simulink model "uz_threephase_VSD_transformation"  (R2021b)
settings: Solver=FixedStepAuto  StartTime=0.0  StopTime=inf  RelTol=1e-3
libraries: hdlsllib x1
settings Model: DataTypeOverride=Off  Creator=ts  LastModifiedBy=valen
settings SolverCC: AlgebraicLoopSolver=TrustRegion  AutoInsertRateTranBlk=on
settings DataIOCC: LimitDataPoints=on  SaveOutput=off  SaveTime=off
settings OptimizationCC: BlockReduction=off  ConditionallyExecuteInputs=off  DefaultParameterBehavior=Inlined  InheritOutputTypeSmallerThanSingle=on  LifeSpan=inf
settings DebuggingCC: AlgebraicLoopMsg=error  SingleTaskRateTransMsg=error  AllowSymbolicDim=off  StrictBusMsg=ErrorOnBusTreatedAsVector  SFUnexpectedBacktrackingDiag=warning  SFNoUnconditionalDefaultTransitionDiag=warning  SFExecutionAtInitializationDiag=none  SFMachineParentedDataDiag=warning  ArithmeticOperatorsInVariantConditions=warning
settings HardwareCC: ProdBitPerPointer=32  ProdBitPerSizeT=32  ProdBitPerPtrDiffT=32  ProdLargestAtomicFloat=None  ProdIntDivRoundTo=Undefined  ProdEndianess=Unspecified  ProdWordSize=32  ProdHWDeviceType=ASIC/FPGA->ASIC/FPGA  ProdEqTarget=off
settings SFSimCC: SimUseLocalCustomCode=off  CustomCodeUndefinedFunction=UseInterfaceOnly
settings RTWCC: RTWUseLocalCustomCode=off
settings CodeAppCC: StateflowObjectComments=on
settings GRTTargetCC: TargetLangStandard=C89/C90 (ANSI)
settings ConfigComp: CovScope=ReferencedModels  CovMetricSettings=dw  CovSaveCumulativeToWorkspaceVar=on  CovSaveSingleToWorkspaceVar=on  CovExternalEMLEnable=off  CovSFcnEnable=off

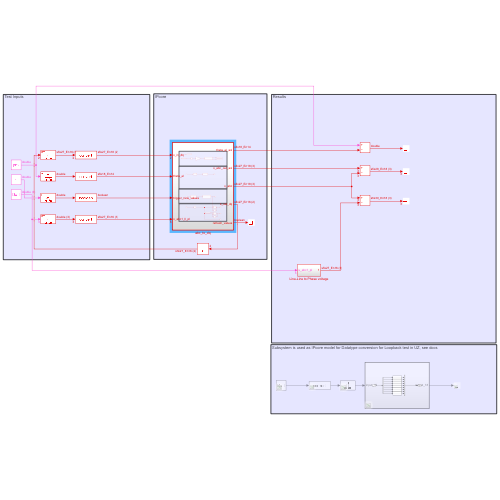
[thumbnail: Simulink's stored preview of the top-level diagram]
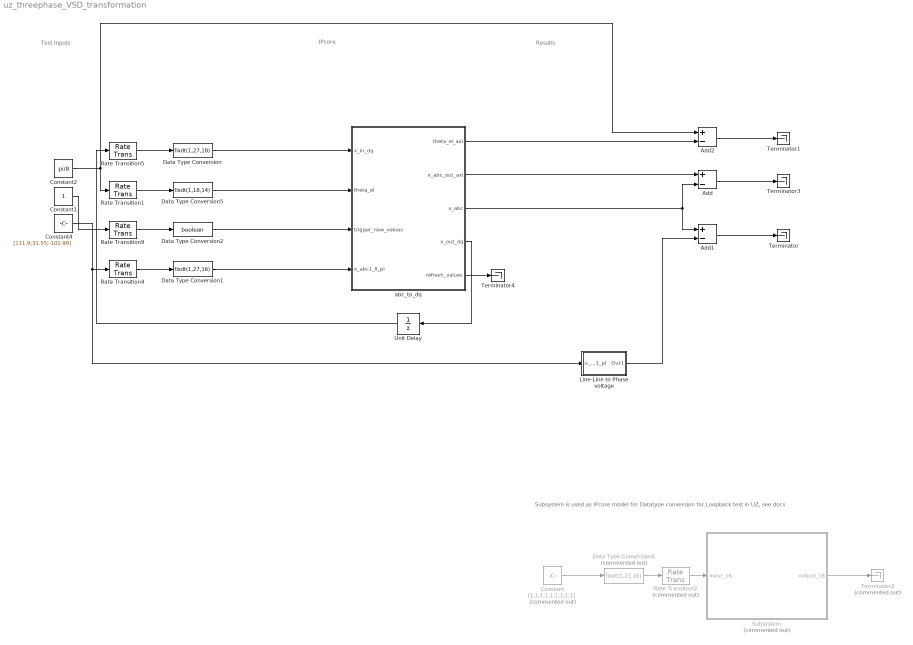
== system uz_threephase_VSD_transformation ==
  note: Subsystem is used as IPcore model for Datatype conversion for Loopback test in UZ, see docs
  note: Results
  note: Test Inputs
  note: IPcore
  Add : Sum  Inputs=+-
  Add1 : Sum  Inputs=+-
  Add2 : Sum  Inputs=+-
  Constant : Constant  Commented=on  Value=[1;1;1;1;1;1;1;1;1]
  Constant1 : Constant
  Constant2 : Constant  Value=pi/8
  Constant4 : Constant  Value=[111.9;31.55;-101.99]
  Data Type Conversion : DataTypeConversion  OutDataTypeStr=fixdt(1,27,18)
  Data Type Conversion1 : DataTypeConversion  OutDataTypeStr=fixdt(1,27,16)
  Data Type Conversion2 : DataTypeConversion  OutDataTypeStr=boolean
  Data Type Conversion5 : DataTypeConversion  OutDataTypeStr=fixdt(1,18,14)
  Data Type Conversion6 : DataTypeConversion  Commented=on  OutDataTypeStr=fixdt(1,27,16)
  Line-Line to Phase voltage : Subsystem
  Rate Transition{1,4..5,9} (4 alike) : RateTransition  OutPortSampleTime=ts_uz_ninephase_VSD_transformation
  Rate Transition2 : RateTransition  Commented=on  OutPortSampleTime=ts_uz_ninephase_VSD_transformation
  Subsystem : Subsystem  Commented=on  TreatAsAtomicUnit=on
  Terminator{,1,3..4} (4 alike) : Terminator
  Terminator2 : Terminator  Commented=on
  Unit Delay : UnitDelay  SampleTime=-1  HasFrameUpgradeWarning=on
  abc_to_dq : Subsystem  TreatAsAtomicUnit=on
  wires:
  Data Type Conversion/1 -> abc_to_dq/1(x_in_dq)
  Data Type Conversion1/1 -> abc_to_dq/4(x_abc1_ll_pl)
  Rate Transition5/1 -> Data Type Conversion/1
  Rate Transition4/1 -> Data Type Conversion1/1
  Data Type Conversion2/1 -> abc_to_dq/3(trigger_new_values)
  Rate Transition9/1 -> Data Type Conversion2/1
  Constant1/1 -> Rate Transition9/1
  Data Type Conversion5/1 -> abc_to_dq/2(theta_el)
  Rate Transition1/1 -> Data Type Conversion5/1
  abc_to_dq/4(x_out_dq) -> Unit Delay/1
  Constant2/1 -> Add2/1, Rate Transition1/1
  abc_to_dq/3(x_abc) -> Add1/1, Add/2
  abc_to_dq/2(x_abc_out_axi) -> Add/1
  Add1/1 -> Terminator/1
  abc_to_dq/1(theta_el_axi) -> Add2/2
  Add2/1 -> Terminator1/1
  Constant4/1 -> Line-Line to Phase voltage/1(u_abc1_pl), Rate Transition4/1
  Add/1 -> Terminator3/1
  Unit Delay/1 -> Rate Transition5/1
  Line-Line to Phase voltage/1(Out1) -> Add1/2
  Subsystem/1(output_18) -> Terminator2/1
  Constant/1 -> Data Type Conversion6/1
  Data Type Conversion6/1 -> Rate Transition2/1
  Rate Transition2/1 -> Subsystem/1(input_16)
  abc_to_dq/5(refresh_values) -> Terminator4/1

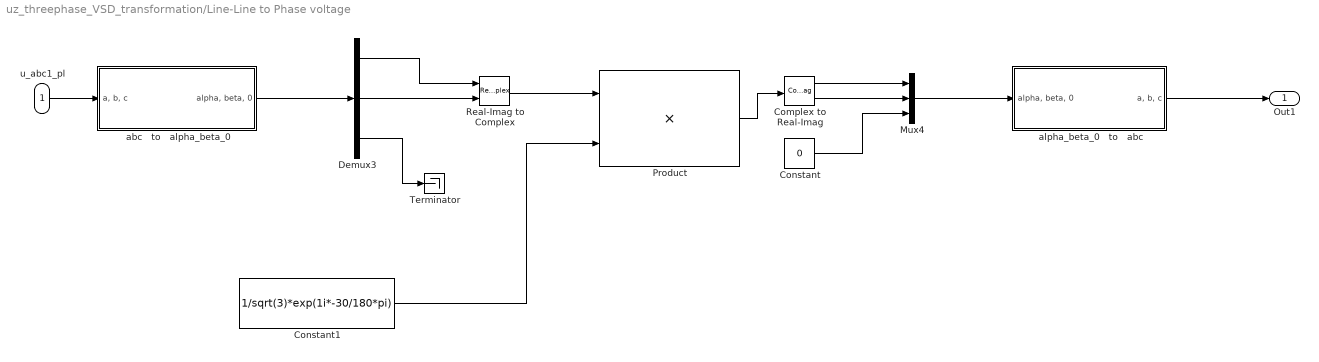
== system uz_threephase_VSD_transformation/Line-Line to Phase voltage ==
  u_abc1_pl : Inport
  Complex to Real-Imag : ComplexToRealImag
  Constant : Constant  Value=0  OutDataTypeStr=fixdt(1,27,16)  SampleTime=-1
  Constant1 : Constant  Value=1/sqrt(3)*exp(1i*-30/180*pi)  OutDataTypeStr=fixdt(1,18,16)  SampleTime=-1
  Demux3 : Demux  Outputs=3
  Mux4 : Mux  Inputs=3
  Product : Product  OutDataTypeStr=fixdt(1,27,16)
  Real-Imag to Complex : RealImagToComplex
  Terminator : Terminator
  abc   to   alpha_beta_0 : Subsystem
  alpha_beta_0   to   abc : Subsystem
  Out1 : Outport
  wires:
  Demux3/2 -> Real-Imag to Complex/2
  Complex to Real-Imag/1 -> Mux4/1
  Mux4/1 -> alpha_beta_0   to   abc/1("alpha, beta, 0  ")
  Product/1 -> Complex to Real-Imag/1
  Real-Imag to Complex/1 -> Product/1
  Demux3/1 -> Real-Imag to Complex/1
  Complex to Real-Imag/2 -> Mux4/2
  Constant/1 -> Mux4/3
  u_abc1_pl/1 -> abc   to   alpha_beta_0/1("a, b, c")
  Demux3/3 -> Terminator/1
  abc   to   alpha_beta_0/1("alpha, beta, 0 ") -> Demux3/1
  alpha_beta_0   to   abc/1("a, b, c") -> Out1/1
  Constant1/1 -> Product/2

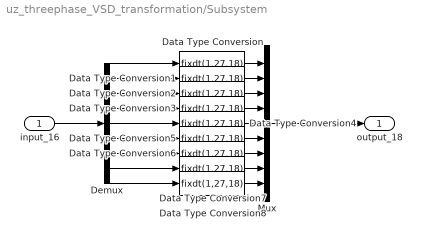
== system uz_threephase_VSD_transformation/Subsystem ==
  input_16 : Inport
  Data Type Conversion{,1..8} (9 alike) : DataTypeConversion  OutDataTypeStr=fixdt(1,27,18)
  Demux : Demux  Outputs=9
  Mux : Mux  Inputs=9
  output_18 : Outport
  wires:
  input_16/1 -> Demux/1
  Demux/1 -> Data Type Conversion/1
  Demux/2 -> Data Type Conversion1/1
  Demux/3 -> Data Type Conversion2/1
  Demux/6 -> Data Type Conversion5/1
  Demux/5 -> Data Type Conversion4/1
  Demux/4 -> Data Type Conversion3/1
  Demux/7 -> Data Type Conversion6/1
  Demux/8 -> Data Type Conversion7/1
  Demux/9 -> Data Type Conversion8/1
  Data Type Conversion/1 -> Mux/1
  Data Type Conversion1/1 -> Mux/2
  Data Type Conversion2/1 -> Mux/3
  Data Type Conversion3/1 -> Mux/4
  Data Type Conversion4/1 -> Mux/5
  Data Type Conversion5/1 -> Mux/6
  Data Type Conversion6/1 -> Mux/7
  Data Type Conversion7/1 -> Mux/8
  Data Type Conversion8/1 -> Mux/9
  Mux/1 -> output_18/1

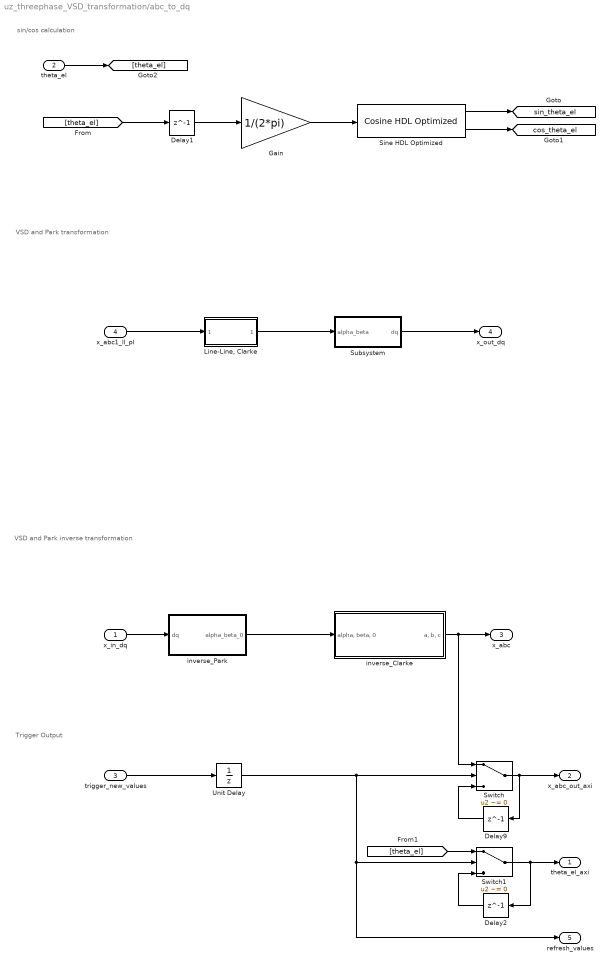
== system uz_threephase_VSD_transformation/abc_to_dq ==
  note: Trigger Output
  note: VSD and Park inverse transformation
  note: VSD and Park transformation
  note: sin/cos calculation
  x_in_dq : Inport
  theta_el : Inport  Port=2
  trigger_new_values : Inport  Port=3
  x_abc1_ll_pl : Inport  Port=4
  Delay1 : Delay  DelayLength=1
  Delay2 : Delay  DelayLength=1
  Delay9 : Delay  DelayLength=1
  Gain : Gain  Gain=1/(2*pi)  OutDataTypeStr=fixdt(1,18,16)
  "Line-Line, Clarke" : Subsystem
  Sine HDL Optimized : hdlsllib/Lookup Tables/Cosine HDL Optimized  OutputFormula=sin(2*pi*u) and cos(2*pi*u)  NumDataPoints=256  TableDataTypeStr=fixdt(0,17,16)  SimulateLUTROMDelay=off
      settings: SourceProductBaseCode=SL
  Subsystem : Subsystem
  Switch : Switch  Criteria=u2 ~= 0
  Switch1 : Switch  Criteria=u2 ~= 0
  Unit Delay : UnitDelay  SampleTime=-1  HasFrameUpgradeWarning=on
  inverse_Clarke : Subsystem
  inverse_Park : Subsystem
  theta_el_axi : Outport
  x_abc_out_axi : Outport  Port=2
  x_abc : Outport  Port=3
  x_out_dq : Outport  Port=4
  refresh_values : Outport  Port=5
  tag scope: cos_theta_el=global, sin_theta_el=global
  wires:
  "Line-Line, Clarke"/1(alpha_beta) -> Subsystem/1(alpha_beta)
  Delay9/1 -> Switch/3
  trigger_new_values/1 -> Unit Delay/1
  Switch/1 -> x_abc_out_axi/1, Delay9/1
  Delay1/1 -> Gain/1
  x_abc1_ll_pl/1 -> "Line-Line, Clarke"/1(u_abc1_pl)
  Gain/1 -> Sine HDL Optimized/1
  Sine HDL Optimized/1 -> [sin_theta_el]
  Sine HDL Optimized/2 -> [cos_theta_el]
  Delay2/1 -> Switch1/3
  Switch1/1 -> theta_el_axi/1, Delay2/1
  Unit Delay/1 -> refresh_values/1, Switch1/2, Switch/2
  Subsystem/1(dq) -> x_out_dq/1
  theta_el/1 -> [theta_el]
  [theta_el] -> Delay1/1
  [theta_el] -> Switch1/1
  inverse_Park/1(alpha_beta_0) -> inverse_Clarke/1("alpha, beta, 0  ")
  x_in_dq/1 -> inverse_Park/1(dq)
  inverse_Clarke/1("a, b, c") -> Switch/1, x_abc/1

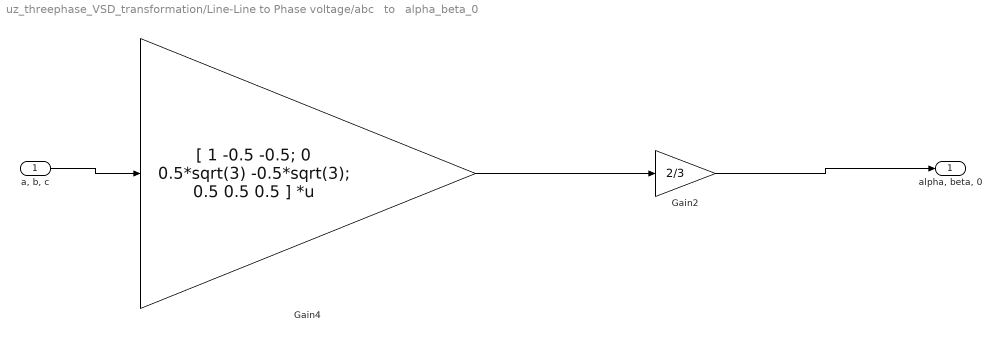
== system uz_threephase_VSD_transformation/Line-Line to Phase voltage/abc   to   alpha_beta_0 ==
  "a, b, c" : Inport  PortDimensions=3
  Gain2 : Gain  Gain=2/3  ParamDataTypeStr=fixdt(1,18,16)  SaturateOnIntegerOverflow=on  OutDataTypeStr=Inherit: Same as input
  Gain4 : Gain  Gain="[ 1   -0.5   -0.5; 0   0.5*sqrt(3)   -0.5*sqrt(3); 0.5  0.5  0.5 ]"  Multiplication=Matrix(K*u) (u vector)  ParamDataTypeStr=fixdt(1,18,16)  OutDataTypeStr=fixdt(1,27,16)  SaturateOnIntegerOverflow=on
  "alpha, beta, 0 " : Outport
  wires:
  Gain2/1 -> "alpha, beta, 0 "/1
  "a, b, c"/1 -> Gain4/1
  Gain4/1 -> Gain2/1

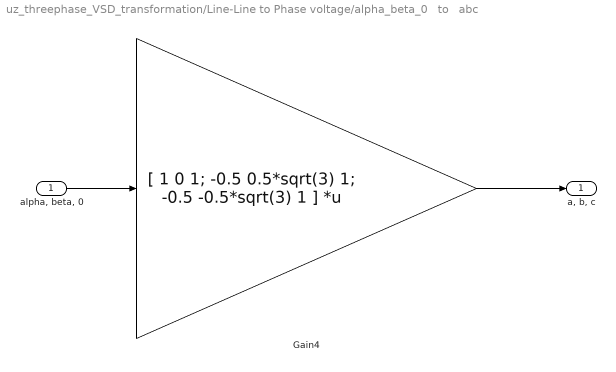
== system uz_threephase_VSD_transformation/Line-Line to Phase voltage/alpha_beta_0   to   abc ==
  "alpha, beta, 0  " : Inport  PortDimensions=3
  Gain4 : Gain  Gain="[ 1 0 1; -0.5   0.5*sqrt(3)  1; -0.5 -0.5*sqrt(3) 1 ]"  Multiplication=Matrix(K*u) (u vector)  ParamDataTypeStr=fixdt(1,18,16)  SaturateOnIntegerOverflow=on  OutDataTypeStr=Inherit: Same as input
  "a, b, c" : Outport
  wires:
  Gain4/1 -> "a, b, c"/1
  "alpha, beta, 0  "/1 -> Gain4/1

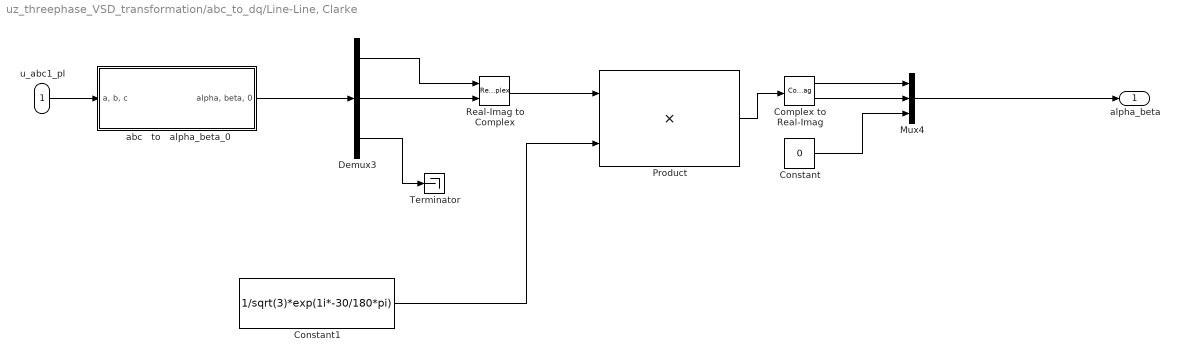
== system uz_threephase_VSD_transformation/abc_to_dq/Line-Line, Clarke ==
  u_abc1_pl : Inport
  Complex to Real-Imag : ComplexToRealImag
  Constant : Constant  Value=0  OutDataTypeStr=fixdt(1,27,16)  SampleTime=-1
  Constant1 : Constant  Value=1/sqrt(3)*exp(1i*-30/180*pi)  OutDataTypeStr=fixdt(1,18,16)  SampleTime=-1
  Demux3 : Demux  Outputs=3
  Mux4 : Mux  Inputs=3
  Product : Product  OutDataTypeStr=fixdt(1,27,16)
  Real-Imag to Complex : RealImagToComplex
  Terminator : Terminator
  abc   to   alpha_beta_0 : Subsystem
  alpha_beta : Outport
  wires:
  Demux3/2 -> Real-Imag to Complex/2
  Complex to Real-Imag/1 -> Mux4/1
  Product/1 -> Complex to Real-Imag/1
  Real-Imag to Complex/1 -> Product/1
  Demux3/1 -> Real-Imag to Complex/1
  Complex to Real-Imag/2 -> Mux4/2
  Constant/1 -> Mux4/3
  u_abc1_pl/1 -> abc   to   alpha_beta_0/1("a, b, c")
  Demux3/3 -> Terminator/1
  abc   to   alpha_beta_0/1("alpha, beta, 0 ") -> Demux3/1
  Mux4/1 -> alpha_beta/1
  Constant1/1 -> Product/2

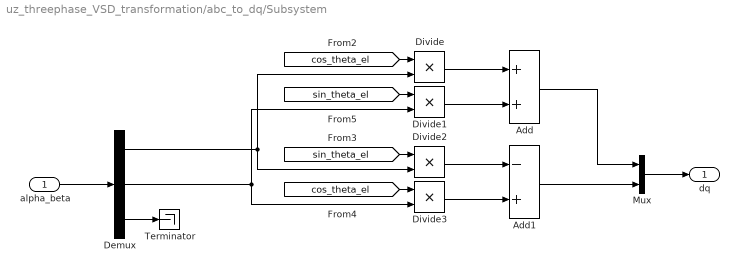
== system uz_threephase_VSD_transformation/abc_to_dq/Subsystem ==
  alpha_beta : Inport
  Add : Sum  OutDataTypeStr=fixdt(1,27,16)
  Add1 : Sum  Inputs=-+  OutDataTypeStr=fixdt(1,27,16)
  Demux : Demux  Outputs=3
  Divide{,1..3} (4 alike) : Product  Inputs=**  OutDataTypeStr=fixdt(1,27,16)
  Mux : Mux  Inputs=2
  Terminator : Terminator
  dq : Outport
  wires:
  Demux/2 -> Divide1/2, Divide3/2
  [cos_theta_el] -> Divide3/1
  Divide3/1 -> Add1/2
  Divide2/1 -> Add1/1
  Divide/1 -> Add/1
  [sin_theta_el] -> Divide2/1
  [cos_theta_el] -> Divide/1
  Demux/1 -> Divide/2, Divide2/2
  Divide1/1 -> Add/2
  [sin_theta_el] -> Divide1/1
  Add/1 -> Mux/1
  Add1/1 -> Mux/2
  Demux/3 -> Terminator/1
  alpha_beta/1 -> Demux/1
  Mux/1 -> dq/1

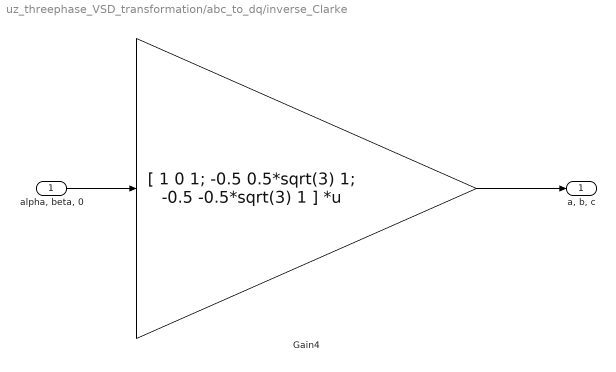
== system uz_threephase_VSD_transformation/abc_to_dq/inverse_Clarke ==
  "alpha, beta, 0  " : Inport  PortDimensions=3
  Gain4 : Gain  Gain="[ 1 0 1; -0.5   0.5*sqrt(3)  1; -0.5 -0.5*sqrt(3) 1 ]"  Multiplication=Matrix(K*u) (u vector)  ParamDataTypeStr=fixdt(1,18,16)  SaturateOnIntegerOverflow=on  OutDataTypeStr=Inherit: Same as input
  "a, b, c" : Outport
  wires:
  Gain4/1 -> "a, b, c"/1
  "alpha, beta, 0  "/1 -> Gain4/1

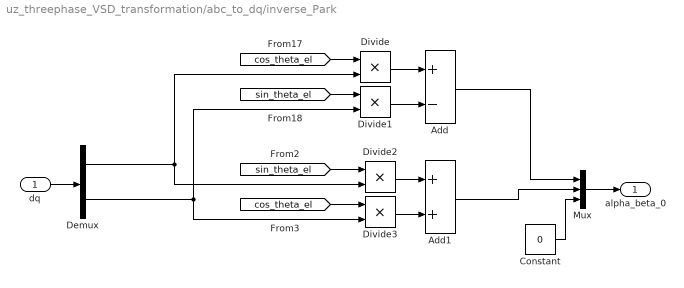
== system uz_threephase_VSD_transformation/abc_to_dq/inverse_Park ==
  dq : Inport
  Add : Sum  Inputs=+-  OutDataTypeStr=fixdt(1,27,18)
  Add1 : Sum  OutDataTypeStr=fixdt(1,27,18)
  Constant : Constant  Value=0  OutDataTypeStr=Inherit: Inherit via back propagation  SampleTime=-1
  Demux : Demux  Outputs=2
  Divide{,1..3} (4 alike) : Product  Inputs=**  OutDataTypeStr=fixdt(1,27,18)
  Mux : Mux  Inputs=3
  alpha_beta_0 : Outport
  wires:
  Divide1/1 -> Add/2
  Divide2/1 -> Add1/1
  Demux/1 -> Divide/2, Divide2/2
  Divide/1 -> Add/1
  Demux/2 -> Divide1/2, Divide3/2
  [cos_theta_el] -> Divide3/1
  [sin_theta_el] -> Divide2/1
  Add1/1 -> Mux/2
  [cos_theta_el] -> Divide/1
  [sin_theta_el] -> Divide1/1
  Divide3/1 -> Add1/2
  Add/1 -> Mux/1
  dq/1 -> Demux/1
  Mux/1 -> alpha_beta_0/1
  Constant/1 -> Mux/3

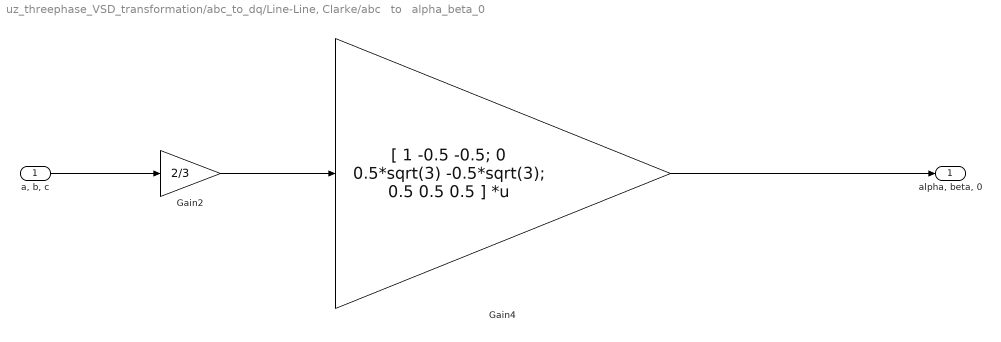
== system uz_threephase_VSD_transformation/abc_to_dq/Line-Line, Clarke/abc   to   alpha_beta_0 ==
  "a, b, c" : Inport  PortDimensions=3
  Gain2 : Gain  Gain=2/3  ParamDataTypeStr=fixdt(1,18,16)  SaturateOnIntegerOverflow=on  OutDataTypeStr=Inherit: Same as input
  Gain4 : Gain  Gain="[ 1   -0.5   -0.5; 0   0.5*sqrt(3)   -0.5*sqrt(3); 0.5  0.5  0.5 ]"  Multiplication=Matrix(K*u) (u vector)  ParamDataTypeStr=fixdt(1,18,16)  OutDataTypeStr=fixdt(1,27,16)  SaturateOnIntegerOverflow=on
  "alpha, beta, 0 " : Outport
  wires:
  Gain4/1 -> "alpha, beta, 0 "/1
  "a, b, c"/1 -> Gain2/1
  Gain2/1 -> Gain4/1
